simulink model "verify_Resident_Data_mdl"  (R2018b)
settings: Solver=ode45  StartTime=0  StopTime=2*24*3600  MaxStep=10  RelTol=1e-3  EnableMultiTasking=on
libraries: simulink x3, carnot x1
settings Model: Creator=drhf  LastModifiedBy=drhf
settings DataIOCC: SaveFormat=Array  SignalLoggingSaveFormat=ModelDataLogs
settings OptimizationCC: ExpressionDepthLimit=2147483647  LifeSpan=inf
settings DebuggingCC: UnderspecifiedInitializationDetection=Classic  MergeDetectMultiDrivingBlocksExec=none  SolverPrmCheckMsg=warning  FcnCallInpInsideContextMsg=warning  StateNameClashWarn=warning  SFUnexpectedBacktrackingDiag=warning  SFNoUnconditionalDefaultTransitionDiag=warning  SFExecutionAtInitializationDiag=none
settings HardwareCC: ProdBitPerPointer=32  ProdBitPerSizeT=32  ProdBitPerPtrDiffT=32  ProdLargestAtomicFloat=None  ProdIntDivRoundTo=Undefined  ProdEndianess=Unspecified  ProdWordSize=32  ProdHWDeviceType=32-bit Generic
settings ModelReferenceCC: PropagateSignalLabelsOutOfModel=off
settings SFSimCC: SimUseLocalCustomCode=off
settings RTWCC: RTWUseLocalCustomCode=off
settings CodeAppCC: StateflowObjectComments=on
settings GRTTargetCC: TargetLangStandard=C89/C90 (ANSI)  GeneratePreprocessorConditionals=Disable all  CombineOutputUpdateFcns=off  GRTInterface=on
settings ConfigComp: CovMetricSettings=dw  CovHtmlReporting=on  CovSaveCumulativeToWorkspaceVar=on  CovSaveSingleToWorkspaceVar=on  CovExternalEMLEnable=off

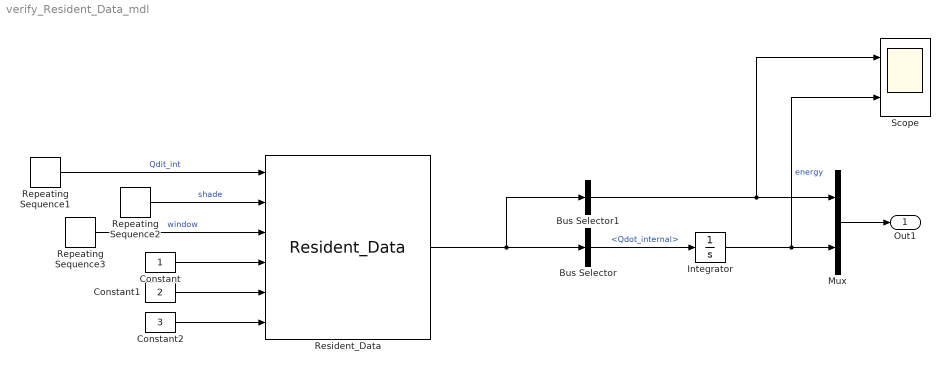
== system verify_Resident_Data_mdl ==
  Bus Selector : BusSelector  OutputSignals=Qdot_internal
  Bus Selector1 : BusSelector  OutputSignals=Sunshade,OpenWindow,CalculateAirComposition,Massflow_CO2,Massflow_H2O,Massflow_VOC  OutputAsBus=on
  Constant : Constant
  Constant1 : Constant  Value=2
  Constant2 : Constant  Value=3
  Integrator : Integrator
  Mux : Mux  Inputs=2
  Repeating Sequence1 : simulink/Sources/Repeating Sequence  rep_seq_t="[0  12 24]*3600"  rep_seq_y=[100 500 100]
  Repeating Sequence2 : simulink/Sources/Repeating Sequence  rep_seq_t="[0  12 24]*3600"  rep_seq_y=[0 1 0]
  Repeating Sequence3 : simulink/Sources/Repeating Sequence  rep_seq_t=[0 8 9 10 12 18 19 20 24]*3600  rep_seq_y=[0 0 1 1 0 0 1 1 0]
  Resident_Data : carnot/Load/Houses/Resident_Data  CalcAirComp=on
      settings: SourceProductName=Carnot
  Scope : Scope  NumInputPorts=2
  Out1 : Outport
  wires:
  Integrator/1 -> Scope/2, Mux/2  "energy"
  Resident_Data/1 -> Bus Selector1/1, Bus Selector/1
  Bus Selector/1 -> Integrator/1  "<Qdot_internal>"
  Mux/1 -> Out1/1
  Bus Selector1/1 -> Scope/1, Mux/1
  Constant2/1 -> Resident_Data/6
  Constant1/1 -> Resident_Data/5
  Repeating Sequence3/1 -> Resident_Data/3  "window"
  Repeating Sequence1/1 -> Resident_Data/1  "Qdit_int"
  Repeating Sequence2/1 -> Resident_Data/2  "shade"
  Constant/1 -> Resident_Data/4
